simulink model "FullSim_Kalman"  (R2025b)
settings: Solver=ode4  StartTime=0.0  StopTime=100  FixedStep=0.01  RelTol=1e-3
values from neighbouring files (symbols this model uses):
  psi_op = pi/2    (= 1.57079632679)    [init_linearization.m]
  theta_op = -10*pi/180    (= -0.174532925199)    [init_linearization.m]
  V_mp_op = (K_yy*m_heli*g*cos(theta_op)*l_cm)/(K_yy*K_pp-K_yp*K_py)    [init_linearization.m]
  V_my_op = (K_yp*V_mp_op)/K_yy    [init_linearization.m]
  w_psi_op = 0    [init_linearization.m]
  w_theta_op = 0    [init_linearization.m]
libraries: realtime_pacer_lib x1
settings Model: Creator=bulve  LastModifiedBy=Torstein

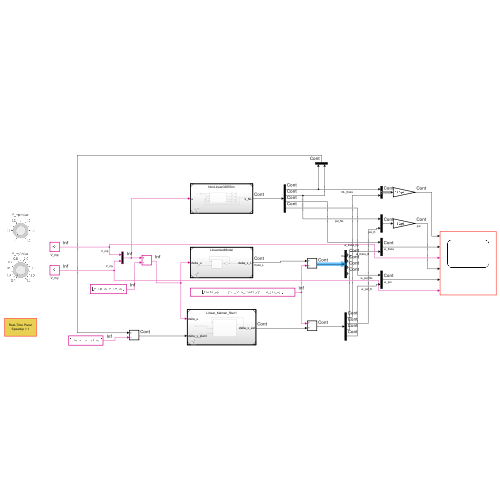
[thumbnail: Simulink's stored preview of the top-level diagram]
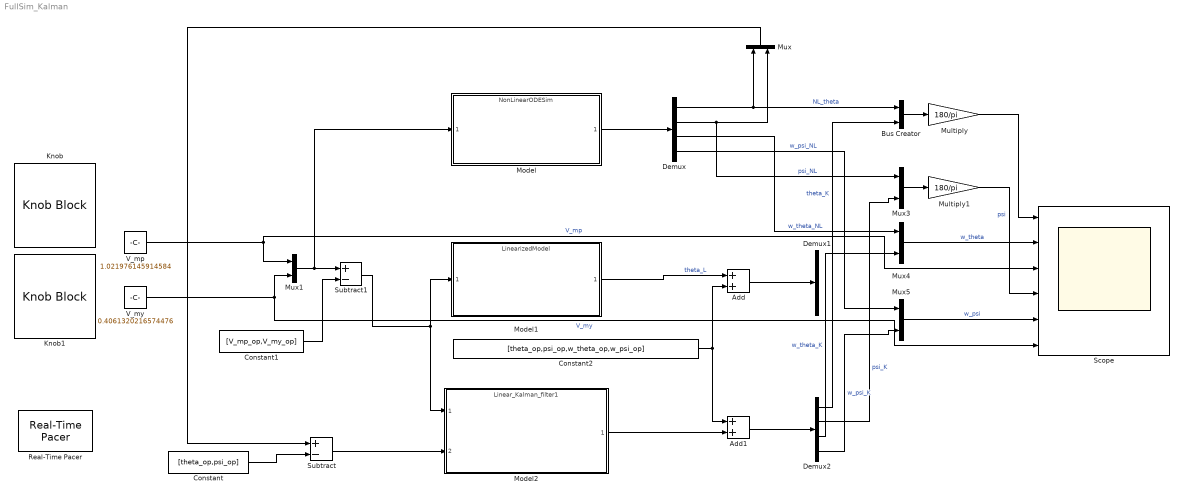
== system FullSim_Kalman ==
  Add : Sum
  Add1 : Sum
  Bus Creator : BusCreator  Inputs=2
  Constant : Constant  Value=[theta_op,psi_op]
  Constant1 : Constant  Value=[V_mp_op,V_my_op]
  Constant2 : Constant  Value=[theta_op,psi_op,w_theta_op,w_psi_op]
  Demux : Demux
  Demux1 : Demux
  Demux2 : Demux
  Knob : KnobBlock  ScaleMin=1  ScaleMax=1.5
  Knob1 : KnobBlock  ScaleMin=0.4  ScaleMax=1.3
  Model : ModelReference  ModelNameDialog=NonLinearODESim.slx  SimulationMode=Normal  ModelReferenceVersion=1.13
  Model1 : ModelReference  ModelNameDialog=LinearizedModel.slx  SimulationMode=Normal  ModelReferenceVersion=1.17
  Model2 : ModelReference  ModelNameDialog=Linear_Kalman_filter1.slx  SimulationMode=Normal  ModelReferenceVersion=1.13
  Multiply : Gain  Gain=180/pi
  Multiply1 : Gain  Gain=180/pi
  Mux{,1,3..5} (5 alike) : Mux  Inputs=2
  Real-Time Pacer : realtime_pacer_lib/Real-Time Pacer  simTimePerRealTime=1
  Scope : Scope  NumInputPorts=6
      settings: ActiveDisplayYMinimum=-16.875  ActiveDisplayYMaximum=51.875
  Subtract : Sum  Inputs=+-
  Subtract1 : Sum  Inputs=+-
  V_mp : Constant  Value=1.021976145914584
  V_my : Constant  Value=0.4061320216574476
  wires:
  Constant/1 -> Subtract/2
  Mux/1 -> Subtract/1
  Mux1/1 -> Subtract1/1, Model/1
  Constant1/1 -> Subtract1/2
  Subtract/1 -> Model2/2
  Model1/1 -> Add/1  "theta_L"
  Constant2/1 -> Add1/1, Add/2
  Model2/1 -> Add1/2
  Add/1 -> Demux1/1
  Add1/1 -> Demux2/1
  Demux/1 -> Bus Creator/1, Mux/1  "NL_theta"
  Demux/2 -> Mux3/1, Mux/2  "psi_NL"
  Demux2/1 -> Bus Creator/2  "theta_K"
  Demux2/2 -> Mux3/2  "psi_K"
  Demux/3 -> Mux4/1  "w_theta_NL"
  Demux2/3 -> Mux4/2  "w_theta_K"
  Demux/4 -> Mux5/1  "w_psi_NL"
  Demux2/4 -> Mux5/2  "w_psi_K"
  Mux3/1 -> Multiply1/1
  Multiply/1 -> Scope/1
  Model/1 -> Demux/1
  Subtract1/1 -> Model1/1, Model2/1
  V_my/1 -> Mux1/2, Scope/6  "V_my"
  V_mp/1 -> Scope/3, Mux1/1  "V_mp"
  Bus Creator/1 -> Multiply/1
  Multiply1/1 -> Scope/4  "psi"
  Mux4/1 -> Scope/2  "w_theta"
  Mux5/1 -> Scope/5  "w_psi"
